simulink model "fir_simple"  (R2024b)
settings: Solver=FixedStepDiscrete  StartTime=0.0  StopTime=0.99987  RelTol=1e-3
undefined symbols (not defined in the file or in its folder): b
Description:
  | Symmetric FIR Filter
  | This example shows how to use HDL Coder(TM) to check, generate,
  | and verify HDL for a fixed-point symmetric FIR filter.
settings Model: DataTypeOverride=Off  Creator=adubu  LastModifiedBy=adubu
settings SolverCC: AlgebraicLoopSolver=TrustRegion
settings DataIOCC: ExternalInput=u  LimitDataPoints=on  LoadExternalInput=on  SaveOutput=off  SaveTime=off  SignalLoggingName=logsOut
settings OptimizationCC: BlockReduction=off  BooleanDataType=off  ConditionallyExecuteInputs=off  DefaultParameterBehavior=Inlined  InlineInvariantSignals=on  EnhancedBackFolding=on  PassReuseOutputArgsAs=Individual arguments  ExpressionDepthLimit=2147483647  ZeroExternalMemoryAtStartup=off  ZeroInternalMemoryAtStartup=off  InitFltsAndDblsToZero=on  BufferReusableBoundary=off  OptimizeBlockOrder=speed  DifferentSizesBufferReuse=on  OptimizationCustomize=off  EfficientTunableParamExpr=on
settings DebuggingCC: AlgebraicLoopMsg=error  SaveWithParameterizedLinksMsg=none  UnderspecifiedInitializationDetection=Classic  MergeDetectMultiDrivingBlocksExec=none  CheckExecutionContextPreStartOutputMsg=on  SignalResolutionControl=TryResolveAllWithWarning  MultiTaskDSMMsg=warning  MultiTaskCondExecSysMsg=none  SingleTaskRateTransMsg=error  IntegerOverflowMsg=none  ParameterPrecisionLossMsg=none  ParameterTunabilityLossMsg=error  FcnCallInpInsideContextMsg=warning  UnconnectedInputMsg=warning  UnconnectedOutputMsg=warning  UnconnectedLineMsg=warning  BusObjectLabelMismatch=none  AllowSymbolicDim=off  StateNameClashWarn=warning  StrictBusMsg=ErrorOnBusTreatedAsVector  SFUnexpectedBacktrackingDiag=warning  SFNoUnconditionalDefaultTransitionDiag=warning  SFExecutionAtInitializationDiag=none  IntegerSaturationMsg=none  ArithmeticOperatorsInVariantConditions=warning
settings HardwareCC: ProdBitPerPointer=32  ProdBitPerSizeT=32  ProdBitPerPtrDiffT=32  ProdLargestAtomicFloat=None  ProdIntDivRoundTo=Undefined  ProdEndianess=Unspecified  ProdWordSize=32  ProdHWDeviceType=ASIC/FPGA->ASIC/FPGA  TargetBitPerPointer=64  TargetBitPerSizeT=64  TargetBitPerPtrDiffT=64  TargetLongLongMode=on  TargetIntDivRoundTo=Zero  TargetEndianess=LittleEndian  TargetWordSize=64  TargetHWDeviceType=MATLAB Host  ProdEqTarget=off
settings ModelReferenceCC: EnableRefExpFcnMdlSchedulingChecks=on
settings SFSimCC: SimUseLocalCustomCode=off  MATLABDynamicMemAlloc=off  CustomCodeUndefinedFunction=UseInterfaceOnly
settings RTWCC: Description=Embedded Coder  SystemTargetFile=ert.tlc  TemplateMakefile=ert_default_tmf  RTWUseLocalCustomCode=off  GPUComputeCapability=3.5
settings CodeAppCC: ForceParamTrailComments=on  IgnoreCustomStorageClasses=off  OperatorAnnotations=on  SimulinkDataObjDesc=on  SFDataObjDesc=on  InsertBlockDesc=on
settings ERTTargetCC: GenerateSampleERTMain=on  ERTCustomFileTemplate=example_file_process.tlc
settings ConfigComp: CovScope=ReferencedModels  CovMetricSettings=dw  CovSaveCumulativeToWorkspaceVar=on  CovSaveSingleToWorkspaceVar=on  CovExternalEMLEnable=off  CovSFcnEnable=off

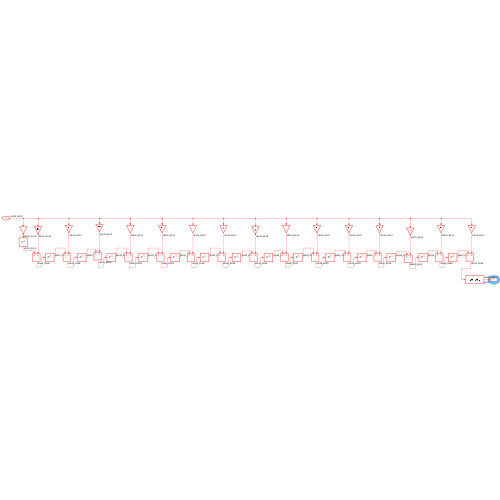
[thumbnail: Simulink's stored preview of the top-level diagram]
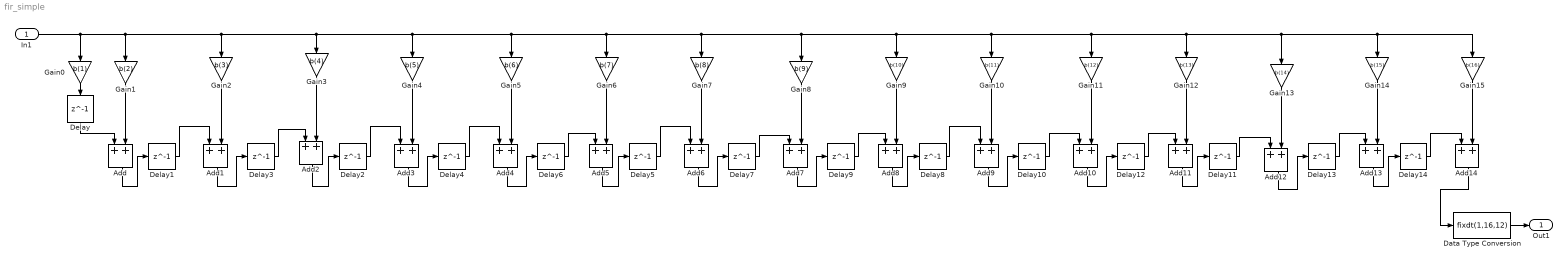
== system fir_simple ==
  In1 : Inport  OutDataTypeStr=fixdt(1,16,12)  PortDimensions=1
  Add{,1..14} (15 alike) : Sum  OutDataTypeStr=fixdt(1,32,26)  AccumDataTypeStr=fixdt(1,32,26)
  Data Type Conversion : DataTypeConversion  OutDataTypeStr=fixdt(1,16,12)  SaturateOnIntegerOverflow=off  RndMeth=Floor
  Delay{,1..14} (15 alike) : Delay  DelayLength=1
  Gain0 : Gain  Gain=b(1)  OutDataTypeStr=fixdt(1,Wc,Dc)
  Gain1 : Gain  Gain=b(2)  OutDataTypeStr=fixdt(1,Wc,Dc)
  Gain10 : Gain  Gain=b(11)  OutDataTypeStr=fixdt(1,Wc,Dc)
  Gain11 : Gain  Gain=b(12)  OutDataTypeStr=fixdt(1,Wc,Dc)
  Gain12 : Gain  Gain=b(13)  OutDataTypeStr=fixdt(1,Wc,Dc)
  Gain13 : Gain  Gain=b(14)  OutDataTypeStr=fixdt(1,Wc,Dc)
  Gain14 : Gain  Gain=b(15)  OutDataTypeStr=fixdt(1,Wc,Dc)
  Gain15 : Gain  Gain=b(16)  OutDataTypeStr=fixdt(1,Wc,Dc)
  Gain2 : Gain  Gain=b(3)  OutDataTypeStr=fixdt(1,Wc,Dc)
  Gain3 : Gain  Gain=b(4)  OutDataTypeStr=fixdt(1,Wc,Dc)
  Gain4 : Gain  Gain=b(5)  OutDataTypeStr=fixdt(1,Wc,Dc)
  Gain5 : Gain  Gain=b(6)  OutDataTypeStr=fixdt(1,Wc,Dc)
  Gain6 : Gain  Gain=b(7)  OutDataTypeStr=fixdt(1,Wc,Dc)
  Gain7 : Gain  Gain=b(8)  OutDataTypeStr=fixdt(1,Wc,Dc)
  Gain8 : Gain  Gain=b(9)  OutDataTypeStr=fixdt(1,Wc,Dc)
  Gain9 : Gain  Gain=b(10)  OutDataTypeStr=fixdt(1,Wc,Dc)
  Out1 : Outport  OutDataTypeStr=fixdt(1,16,12)
  wires:
  Gain0/1 -> Delay/1
  Add/1 -> Delay1/1
  In1/1 -> Gain1/1, Gain2/1, Gain4/1, Gain5/1, Gain7/1, Gain8/1, Gain9/1, Gain10/1, Gain11/1, Gain12/1, Gain13/1, Gain15/1, Gain14/1, Gain6/1, Gain3/1, Gain0/1
  Delay/1 -> Add/1
  Gain2/1 -> Add1/2
  Add1/1 -> Delay3/1
  Delay1/1 -> Add1/1
  Gain3/1 -> Add2/2
  Add2/1 -> Delay2/1
  Delay2/1 -> Add3/1
  Add3/1 -> Delay4/1
  Gain4/1 -> Add3/2
  Delay3/1 -> Add2/1
  Delay4/1 -> Add4/1
  Delay6/1 -> Add5/1
  Add5/1 -> Delay5/1
  Add6/1 -> Delay7/1
  Gain7/1 -> Add6/2
  Add4/1 -> Delay6/1
  Delay5/1 -> Add6/1
  Gain5/1 -> Add4/2
  Delay10/1 -> Add10/1
  Delay7/1 -> Add7/1
  Delay9/1 -> Add8/1
  Gain11/1 -> Add10/2
  Add12/1 -> Delay13/1
  Gain12/1 -> Add11/2
  Gain13/1 -> Add12/2
  Delay11/1 -> Add12/1
  Add10/1 -> Delay12/1
  Gain9/1 -> Add8/2
  Add8/1 -> Delay8/1
  Add9/1 -> Delay10/1
  Add11/1 -> Delay11/1
  Gain10/1 -> Add9/2
  Add7/1 -> Delay9/1
  Delay12/1 -> Add11/1
  Delay8/1 -> Add9/1
  Gain8/1 -> Add7/2
  Delay13/1 -> Add13/1
  Gain14/1 -> Add13/2
  Delay14/1 -> Add14/1
  Gain15/1 -> Add14/2
  Add13/1 -> Delay14/1
  Gain1/1 -> Add/2
  Gain6/1 -> Add5/2
  Data Type Conversion/1 -> Out1/1
  Add14/1 -> Data Type Conversion/1
